simulink model "RBNN_NNT_NN_comparision_exp2"  (R2019a)
settings: Solver=FixedStepAuto  StartTime=0.0  StopTime=inf  FixedStep=0.0000001  RelTol=1e-3
libraries: dspstat3 x4, dsparch4 x2, simulink x1
settings Model: NumberOfSteps=16  Creator=vardhah  LastModifiedBy=vardhah
settings DataIOCC: ReturnWorkspaceOutputs=off
settings DebuggingCC: UnderSpecifiedDimensionMsg=warning  ArithmeticOperatorsInVariantConditions=warning

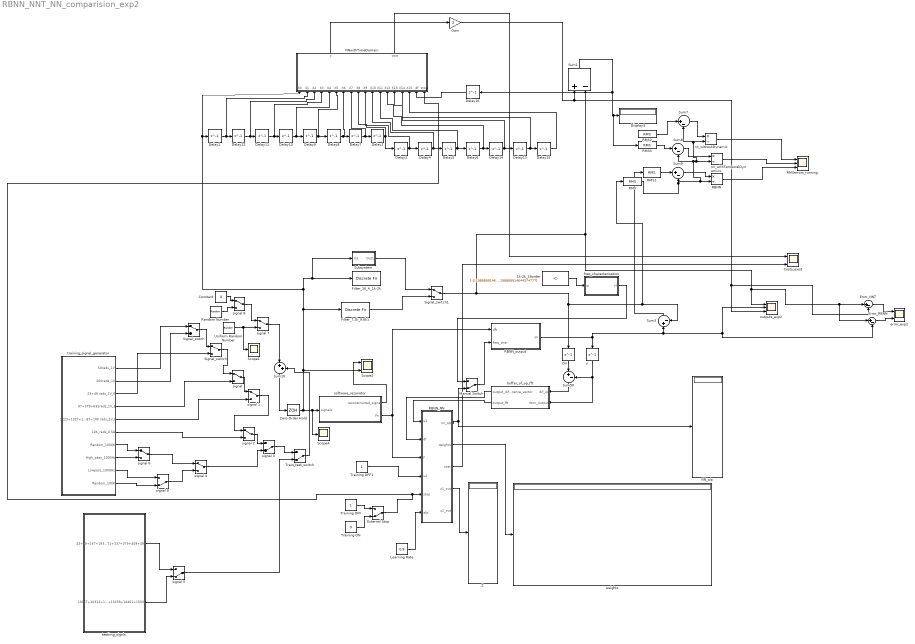
== system RBNN_NNT_NN_comparision_exp2 ==
  1k-2k_16order : Constant  Value=[-0.198889914644374777 0.0882189428518377339 0.0736891495871065116 0.0638368801789635787 0.0566372642221577294 0.0523172683654103132 0.0494565343907736044 0.048157521822162791 0.048157521822162791 0.0494565343907736044 0.0523172683654103132 0.0566372642221577294 0.0638368801789635787 0.0736891495871065116 0.0882189428518377339 -0.198889914644374777]  VectorParams1D=off
  Constant : Constant  Value=0
  Costs_exp2 : Scope  NumInputPorts=2
  Delay{1..16} (16 alike) : Delay  DelayLength=1  InitialCondition=0
  Display3 : Display
  Dn : Delay  DelayLength=1  InitialCondition=0
  Error_NNT : Sum  Inputs=|+-
  Error_RBNN : Sum  Inputs=|+-
  External Stop : ManualSwitch  CurrentSetting=0
  Filter_16_A_1k-2k : DiscreteFir  Tag=BlockMethodSubSystem  Coefficients=[-0.198889914644374777 0.0882189428518377339 0.0736891495871065116 0.0638368801789635787 0.0566372642221577294 0.0523172683654103132 0.0494565343907736044 0.048157521822162791 0.048157521822162791 0.0494565343907736044 0.0523172683654103132 0.0566372642221577294 0.0638368801789635787 0.0736891495871065116 0.0882189428518377339 -0.198889914644374777]  InputProcessing=Columns as channels (frame based)
  Filter_7.2k_9.6k1 : DiscreteFir  Tag=BlockMethodSubSystem  Coefficients=[-0.0120785049852322399 -0.0942455273574688279 0.0101245004695954266 0.125460404555770566 0.034165372769331126 -0.1614987160724079 -0.0984930555982914957 0.150982315564688691 0.150982315564688691 -0.0984930555982914957 -0.1614987160724079 0.034165372769331126 0.125460404555770566 0.0101245004695954266 -0.0942455273574688279 -0.0120785049852322399]  InputProcessing=Columns as channels (frame based)
  Gain : Gain  Gain=2
  Learning Rate : Constant  Value=0.9
  Manual Switch : ManualSwitch  CurrentSetting=0  varsize=on
  NN_o/p : Display
  NNwithTimeDomain : MATLAB Function  TreatAsAtomicUnit=on
  RBNN : Product  Inputs=*/
  RBNN_NN : MATLAB Function  TreatAsAtomicUnit=on
  RBNN_output : MATLAB Function  TreatAsAtomicUnit=on
  RMS{,1..3} (4 alike) : dspstat3/RMS  run=on  directionMode=Each column  dimension=1  InputProcessing=Columns as channels (frame based)  reset_popup=None
  RMSerrors_running : Scope  NumInputPorts=3
  Random Number : RandomNumber  Variance=0.1  SampleTime=0.000001
  Scope1 : Scope
  Scope2 : Scope  NumInputPorts=2
  Scope4 : Scope
  Signal_switch : ManualSwitch
  Signal_switch1 : ManualSwitch
  Signal_swtch : ManualSwitch
  Subsystem : Subsystem
  Sum1 : Sum  Inputs=+-
  Sum10 : Sum  Inputs=|++
  Sum{3,7..9,50} (5 alike) : Sum  Inputs=|+-
  Train_test_switch : ManualSwitch  CurrentSetting=0
  Training OFF : Constant
  Training OFF1 : Constant
  Training ON : Constant  Value=0
  Uniform Random Number : UniformRandomNumber  Minimum=-0.05  Maximum=0.05  SampleTime=0.000001
  Z : Display
  Zero-Order Hold : ZeroOrderHold  SampleTime=0.0000001
  buffer_of_op_fft : MATLAB Function  TreatAsAtomicUnit=on
  error_exp2 : Scope  NumInputPorts=2
  freq_characterisation : MATLAB Function  TreatAsAtomicUnit=on
  nn_withTemporalDynamics : Product  Inputs=*/
  nn_withoutDynamic : Product  Inputs=*/
  outputs_exp2 : Scope  NumInputPorts=3
  signal {,1..2,4,6..8} (7 alike) : ManualSwitch
  signal 3 : ManualSwitch  CurrentSetting=0
  signal 5 : ManualSwitch  CurrentSetting=0
  signal 9 : ManualSwitch  CurrentSetting=0
  software_rezonator : MATLAB Function  TreatAsAtomicUnit=on
  testimg_signls : Subsystem
  training_signal_generator : Subsystem
  weights : Display
  y : Delay  DelayLength=1  InitialCondition=0
  wires:
  software_rezonator/1(reconstructed_signal) -> Scope2/1
  software_rezonator/2(Fn) -> RBNN_output/1(dft), RBNN_NN/3(F)
  Dn/1 -> Sum50/1
  y/1 -> buffer_of_op_fft/2(rbnn_output), Sum50/2
  Manual Switch/1 -> RBNN_output/2(freq_char)
  freq_characterisation/1(H) -> Manual Switch/1
  RBNN_NN/1(nn_op) -> Manual Switch/2, NN_o/p/1
  External Stop/1 -> NNwithTimeDomain/18(stop), RBNN_NN/5(stop)
  Training OFF/1 -> External Stop/1
  Training ON/1 -> External Stop/2
  RBNN_NN/3(cost) -> Costs_exp2/2
  RBNN_NN/2(weights) -> weights/1
  RBNN_NN/4(z1_out) -> Z/1
  1k-2k_16order/1 -> freq_characterisation/1(ip)
  Sum50/1 -> buffer_of_op_fft/1(dif_ip)
  buffer_of_op_fft/1(output_difference_vector) -> RBNN_NN/2(df)
  buffer_of_op_fft/2(output_fft) -> RBNN_NN/1(u1)
  Training OFF1/1 -> RBNN_NN/4(u2)
  Signal_switch/1 -> "signal "/1
  Signal_swtch/1 -> Signal_switch/1
  "signal "/1 -> signal 1/1
  signal 1/1 -> signal 2/1
  training_signal_generator/4(97+379+631rads_1V_E) -> "signal "/2
  training_signal_generator/1(50rads_1V) -> Signal_swtch/1
  training_signal_generator/2(200rads_1V) -> Signal_swtch/2
  training_signal_generator/3(23+46 rads_1V_E) -> Signal_switch/2
  training_signal_generator/5(1223+1327+1637+1787+10K rads_1V_E) -> signal 1/2
  training_signal_generator/6(10K_rads_0.5A) -> signal 2/2
  signal 2/1 -> signal 3/1
  NNwithTimeDomain/1(y) -> Gain/1
  Delay16/1 -> NNwithTimeDomain/17(df)
  Delay4/1 -> NNwithTimeDomain/11(X10), Delay5/1
  Delay6/1 -> Delay14/1, NNwithTimeDomain/13(X12)
  Delay5/1 -> NNwithTimeDomain/12(X11), Delay6/1
  NNwithTimeDomain/2(cost) -> Costs_exp2/1
  Delay2/1 -> Delay3/1, NNwithTimeDomain/9(X8)
  Delay15/1 -> NNwithTimeDomain/16(X15)
  Delay13/1 -> NNwithTimeDomain/15(X14), Delay15/1
  Delay14/1 -> NNwithTimeDomain/14(X13), Delay13/1
  Delay10/1 -> NNwithTimeDomain/5(X4), Delay9/1
  Zero-Order Hold/1 -> Scope2/2, Subsystem/1(In1), Filter_16_A_1k-2k/1, NNwithTimeDomain/1(X0), Delay1/1, Filter_7.2k_9.6k1/1, Scope4/1, software_rezonator/1(signalz)
  Delay3/1 -> Delay4/1, NNwithTimeDomain/10(X9)
  Delay7/1 -> Delay2/1, NNwithTimeDomain/8(X7)
  Delay8/1 -> NNwithTimeDomain/7(X6), Delay7/1
  Delay1/1 -> NNwithTimeDomain/2(X1), Delay12/1
  Delay9/1 -> Delay8/1, NNwithTimeDomain/6(X5)
  Delay12/1 -> NNwithTimeDomain/3(X2), Delay11/1
  Delay11/1 -> Delay10/1, NNwithTimeDomain/4(X3)
  Sum1/1 -> RMS3/1, Display3/1, Delay16/1
  signal 4/1 -> signal 3/2
  Filter_7.2k_9.6k1/1 -> Signal_switch1/2
  nn_withoutDynamic/1 -> RMSerrors_running/1
  nn_withTemporalDynamics/1 -> RMSerrors_running/2
  RBNN/1 -> RMSerrors_running/3
  RMS/1 -> Sum7/2, nn_withoutDynamic/2, nn_withTemporalDynamics/2, Sum8/2, RBNN/2, Sum9/2
  Sum3/1 -> RMS1/1
  RMS1/1 -> Sum9/1
  RMS3/1 -> Sum8/1
  Sum8/1 -> nn_withTemporalDynamics/1
  RMS2/1 -> Sum7/1
  Sum7/1 -> nn_withoutDynamic/1
  testimg_signls/1(43+89+167+193+229+271+337+379+409+499) -> signal 5/1
  testimg_signls/2("10067+10313+10987+11299+11491+12161+12451+13259+14461+15031 ") -> signal 5/2
  signal 3/1 -> Train_test_switch/1
  signal 5/1 -> Train_test_switch/2
  Sum9/1 -> RBNN/1
  signal 7/1 -> Sum10/1
  Sum10/1 -> Zero-Order Hold/1
  Train_test_switch/1 -> Sum10/2
  Uniform Random Number/1 -> Scope1/1, signal 7/2
  Constant/1 -> signal 8/1
  signal 8/1 -> signal 7/1
  Random Number/1 -> signal 8/2
  Error_RBNN/1 -> error_exp2/2
  Gain/1 -> Error_NNT/2, outputs_exp2/3, Sum1/1
  Error_NNT/1 -> error_exp2/1
  Signal_switch1/1 -> Sum1/2, Error_RBNN/1, Error_NNT/1, outputs_exp2/1, RMS/1, Sum3/2, Dn/1
  RBNN_output/1(yn) -> Sum3/1, outputs_exp2/2, Error_RBNN/2, y/1
  signal 9/1 -> signal 4/2
  training_signal_generator/7(Random_1000K) -> signal 6/1
  training_signal_generator/8(High_pass_1000Hz) -> signal 6/2
  training_signal_generator/9(Lowpass_1000Hz) -> signal 9/1
  training_signal_generator/10(Random_100K) -> signal 9/2
  signal 6/1 -> signal 4/1
  Learning Rate/1 -> RBNN_NN/6(alp)
  Subsystem/1(Out1) -> Signal_switch1/1

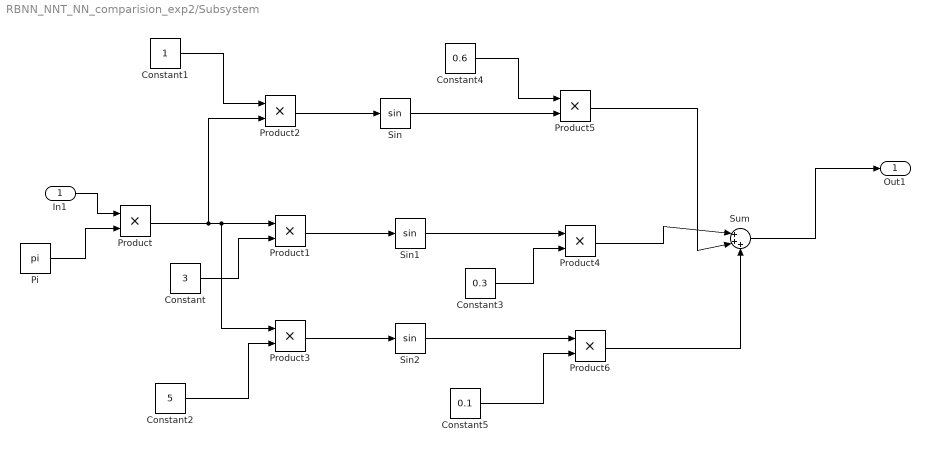
== system RBNN_NNT_NN_comparision_exp2/Subsystem ==
  In1 : Inport
  Constant : Constant  Value=3
  Constant1 : Constant
  Constant2 : Constant  Value=5
  Constant3 : Constant  Value=0.3
  Constant4 : Constant  Value=0.6
  Constant5 : Constant  Value=0.1
  Pi : Constant  Value=pi  OutDataTypeStr=Inherit: Inherit via back propagation
  Product{,1..6} (7 alike) : Product
  Sin : Trigonometry
  Sin1 : Trigonometry
  Sin2 : Trigonometry
  Sum : Sum  Inputs=|+++
  Out1 : Outport
  wires:
  Pi/1 -> Product/2
  In1/1 -> Product/1
  Constant1/1 -> Product2/1
  Product/1 -> Product2/2, Product3/1, Product1/1
  Constant/1 -> Product1/2
  Constant2/1 -> Product3/2
  Product2/1 -> Sin/1
  Product3/1 -> Sin2/1
  Product1/1 -> Sin1/1
  Product5/1 -> Sum/2
  Constant4/1 -> Product5/1
  Product6/1 -> Sum/3
  Constant5/1 -> Product6/2
  Constant3/1 -> Product4/2
  Product4/1 -> Sum/1
  Sin1/1 -> Product4/1
  Sin/1 -> Product5/2
  Sin2/1 -> Product6/1
  Sum/1 -> Out1/1

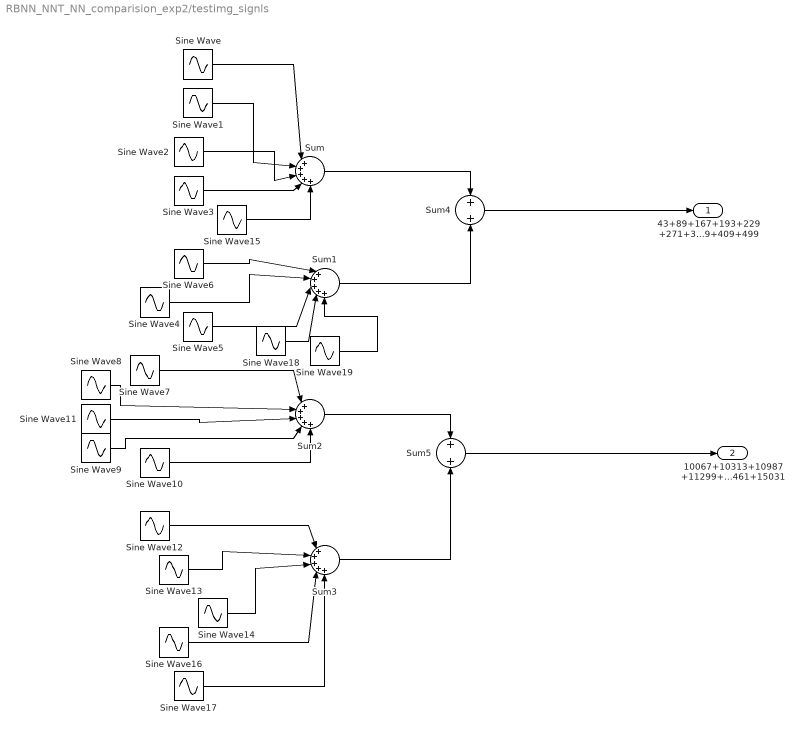
== system RBNN_NNT_NN_comparision_exp2/testimg_signls ==
  Sine Wave : Sin  Amplitude=0.1  Frequency=43  SampleTime=0
  Sine Wave1 : Sin  Amplitude=0.1  Frequency=89  SampleTime=0
  Sine Wave10 : Sin  Amplitude=0.1  Frequency=1491  SampleTime=0
  Sine Wave11 : Sin  Amplitude=0.1  Frequency=1987  SampleTime=0
  Sine Wave12 : Sin  Amplitude=0.1  Frequency=1261  SampleTime=0
  Sine Wave13 : Sin  Amplitude=0.1  Frequency=1451  SampleTime=0
  Sine Wave14 : Sin  Amplitude=0.1  Frequency=3359  SampleTime=0
  Sine Wave15 : Sin  Amplitude=0.1  Frequency=229  SampleTime=0
  Sine Wave16 : Sin  Amplitude=0.1  Frequency=2761  SampleTime=0
  Sine Wave17 : Sin  Amplitude=0.1  Frequency=2931  SampleTime=0
  Sine Wave18 : Sin  Amplitude=0.1  Frequency=409  SampleTime=0
  Sine Wave19 : Sin  Amplitude=0.1  Frequency=499  SampleTime=0
  Sine Wave2 : Sin  Amplitude=0.1  Frequency=167  SampleTime=0
  Sine Wave3 : Sin  Amplitude=0.1  Frequency=193  SampleTime=0
  Sine Wave4 : Sin  Amplitude=0.1  Frequency=337  SampleTime=0
  Sine Wave5 : Sin  Amplitude=0.1  Frequency=379  SampleTime=0
  Sine Wave6 : Sin  Amplitude=0.1  Frequency=271  SampleTime=0
  Sine Wave7 : Sin  Amplitude=0.1  Frequency=1067  SampleTime=0
  Sine Wave8 : Sin  Amplitude=0.1  Frequency=1313  SampleTime=0
  Sine Wave9 : Sin  Amplitude=0.1  Frequency=1299  SampleTime=0
  Sum{,1..3} (4 alike) : Sum  Inputs=|+++++
  Sum4 : Sum
  Sum5 : Sum
  43+89+167+193+229+271+337+379+409+499 : Outport
  "10067+10313+10987+11299+11491+12161+12451+13259+14461+15031 " : Outport  Port=2
  wires:
  Sine Wave4/1 -> Sum1/2
  Sine Wave5/1 -> Sum1/3
  Sine Wave6/1 -> Sum1/1
  Sine Wave7/1 -> Sum2/1
  Sine Wave8/1 -> Sum2/2
  Sine Wave11/1 -> Sum2/3
  Sine Wave9/1 -> Sum2/4
  Sine Wave10/1 -> Sum2/5
  Sine Wave/1 -> Sum/1
  Sine Wave1/1 -> Sum/2
  Sine Wave2/1 -> Sum/3
  Sine Wave3/1 -> Sum/4
  Sine Wave15/1 -> Sum/5
  Sine Wave17/1 -> Sum3/5
  Sine Wave16/1 -> Sum3/4
  Sine Wave14/1 -> Sum3/3
  Sine Wave13/1 -> Sum3/2
  Sine Wave12/1 -> Sum3/1
  Sine Wave18/1 -> Sum1/4
  Sine Wave19/1 -> Sum1/5
  Sum1/1 -> Sum4/2
  Sum/1 -> Sum4/1
  Sum4/1 -> 43+89+167+193+229+271+337+379+409+499/1
  Sum5/1 -> "10067+10313+10987+11299+11491+12161+12451+13259+14461+15031 "/1
  Sum2/1 -> Sum5/1
  Sum3/1 -> Sum5/2

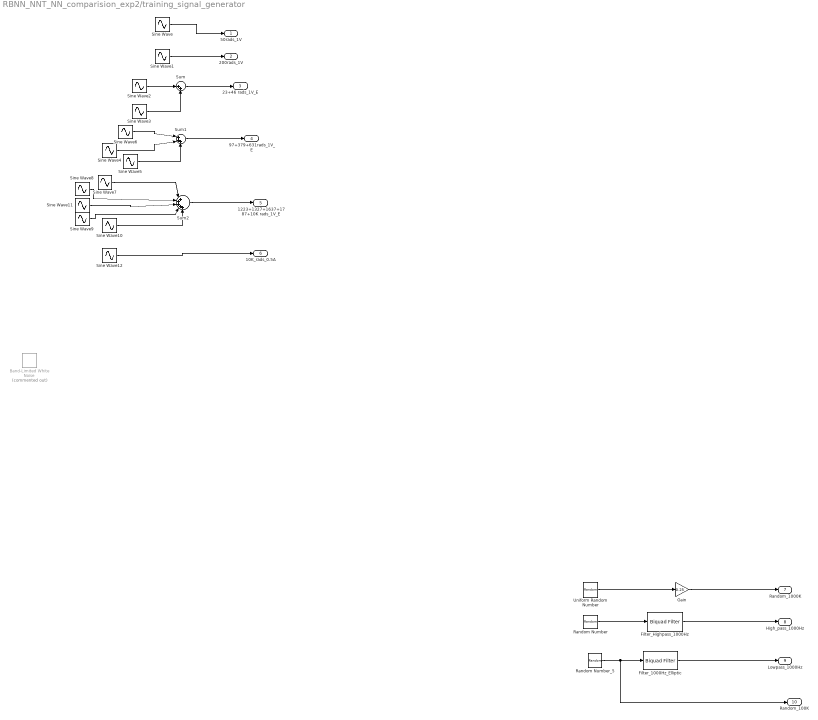
== system RBNN_NNT_NN_comparision_exp2/training_signal_generator ==
  Band-Limited White Noise : simulink/Sources/Band-Limited White Noise  Commented=on  Cov=[0.1]  Ts=0.1  seed=[23341]
  Filter_1000Hz_Elliptic : dsparch4/Biquad Filter  Tag=BlockMethodSubSystem  FilterSource=Dialog parameters  CoeffSource=Specify via dialog  FilterObject=BQF  IIRFiltStruct=Direct form II  BiQuadCoeffs=[1 -1.97632274641133088 1 1 -1.97939835930391728 0.996447647782941925;1 -1.97278944538463175 1 1 -1.97237302925889701 0.987301248342435933;1 -1.95955871016892758 1 1 -1.96235771308246942 0.972660421241710926;1 -1.88453112329299022 1 1 -1.95007892273323602 0.954154972801176005;1 1 0 1 -0.971866907997287366 0]  ScaleValues=[0.156742012624585314;0.548618699418480849;0.254757160374388947;0.035299988916345823;0.064621492680459483;1]  IC=0  ICnum=0  ICden=0  a0Flag=Warning  optimizeScaleValues=on  ScaleValueMode=Specify via input port (g)  InputProcessing=Columns as channels (frame based)  roundingMode=Floor  overflowMode=off  scaleValueFracLength=14  denProdOutputFracLength=30  denAccumFracLength=30  secondMemoryFracLength=15
      settings: SourceProductName=DSP System Toolbox
  Filter_Highpass_1000Hz : dsparch4/Biquad Filter  Tag=BlockMethodSubSystem  FilterSource=Dialog parameters  CoeffSource=Specify via dialog  FilterObject=BQF  IIRFiltStruct=Direct form II  BiQuadCoeffs=[1 -1.9832348135082305 1 1 -1.92871230100246671 0.962722433368264241;1 -1.98583197848424597 1 1 -1.86448430214602556 0.894880266245439038;1 -1.99020937824944788 1 1 -1.81348943480495617 0.839000119522318677;1 -1.99498360843622446 1 1 -1.77690733715439997 0.797591087467987903;1 -1.99863653257112794 1 1 -1.75501257669195576 0.772196386514157451;1 -1 0 1 -0.873867637211059756 0]  ScaleValues=[0.976953385016072651;0.943181897451958351;0.915362881516173843;0.894746706112661938;0.882102920451765637;0.936933818605529933;1]  IC=0  ICnum=0  ICden=0  a0Flag=Warning  optimizeScaleValues=on  ScaleValueMode=Specify via input port (g)  InputProcessing=Columns as channels (frame based)  roundingMode=Floor  overflowMode=off  scaleValueFracLength=14  denProdOutputFracLength=30  denAccumFracLength=30  secondMemoryFracLength=15
      settings: SourceProductName=DSP System Toolbox
  Gain : Gain  Gain=0.25
  Random Number : RandomNumber  Variance=0.5  SampleTime=0.000001
  Random Number_5 : RandomNumber  Variance=0.5  SampleTime=0.000001
  Sine Wave : Sin  Amplitude=0.8  Frequency=50  SampleTime=0
  Sine Wave1 : Sin  Frequency=200  SampleTime=0
  Sine Wave10 : Sin  Amplitude=0.2  Frequency=5000  SampleTime=0
  Sine Wave11 : Sin  Amplitude=0.2  Frequency=1637  SampleTime=0
  Sine Wave12 : Sin  Amplitude=0.5  Frequency=10000  SampleTime=0
  Sine Wave2 : Sin  Amplitude=0.5  Frequency=23  SampleTime=0
  Sine Wave3 : Sin  Amplitude=0.5  Frequency=46  SampleTime=0
  Sine Wave4 : Sin  Amplitude=0.33  Frequency=631  SampleTime=0
  Sine Wave5 : Sin  Amplitude=0.33  Frequency=379  SampleTime=0
  Sine Wave6 : Sin  Amplitude=0.33  Frequency=97  SampleTime=0
  Sine Wave7 : Sin  Amplitude=0.2  Frequency=1223  SampleTime=0
  Sine Wave8 : Sin  Amplitude=0.2  Frequency=1327  SampleTime=0
  Sine Wave9 : Sin  Amplitude=0.2  Frequency=1787  SampleTime=0
  Sum : Sum  Inputs=|++
  Sum1 : Sum  Inputs=|+++
  Sum2 : Sum  Inputs=|+++++
  Uniform Random Number : UniformRandomNumber  Minimum=-2  Maximum=2  SampleTime=0.0000002
  50rads_1V : Outport
  200rads_1V : Outport  Port=2
  23+46 rads_1V_E : Outport  Port=3
  97+379+631rads_1V_E : Outport  Port=4
  1223+1327+1637+1787+10K rads_1V_E : Outport  Port=5
  10K_rads_0.5A : Outport  Port=6
  Random_1000K : Outport  Port=7
  High_pass_1000Hz : Outport  Port=8
  Lowpass_1000Hz : Outport  Port=9
  Random_100K : Outport  Port=10
  wires:
  Sine Wave/1 -> 50rads_1V/1
  Sine Wave1/1 -> 200rads_1V/1
  Sine Wave2/1 -> Sum/1
  Sine Wave3/1 -> Sum/2
  Sum/1 -> 23+46 rads_1V_E/1
  Sine Wave4/1 -> Sum1/2
  Sine Wave5/1 -> Sum1/3
  Sine Wave6/1 -> Sum1/1
  Sum1/1 -> 97+379+631rads_1V_E/1
  Sine Wave7/1 -> Sum2/1
  Sine Wave8/1 -> Sum2/2
  Sine Wave11/1 -> Sum2/3
  Sine Wave9/1 -> Sum2/4
  Sine Wave10/1 -> Sum2/5
  Sum2/1 -> 1223+1327+1637+1787+10K rads_1V_E/1
  Sine Wave12/1 -> 10K_rads_0.5A/1
  Uniform Random Number/1 -> Gain/1
  Gain/1 -> Random_1000K/1
  Random Number/1 -> Filter_Highpass_1000Hz/1
  Filter_Highpass_1000Hz/1 -> High_pass_1000Hz/1
  Filter_1000Hz_Elliptic/1 -> Lowpass_1000Hz/1
  Random Number_5/1 -> Random_100K/1, Filter_1000Hz_Elliptic/1

== matlab function RBNN_NNT_NN_comparision_exp2/RBNN_NN ==
  settings: sampleTime=0.01
  data: u1 input; df input; F input; u2 input; stop input; nn_op output; alp input; weights output; cost output; z1_out output; z2_out output
function [nn_op,weights,cost,z1_out,z2_out]  = NN(u1,df,F,u2,stop,alp)

persistent w1 w2;
persistent vy;
persistent g1 g2;
persistent itr;
persistent J;
persistent del_w1 del_w2;
persistent mult1 mult2 ;
persistent memory_alloc_flag;
persistent n;

%%
%%%%%%----------------------------------------------------------------------------%%%%%
%Hyper-parameter & other tunable part of code

M=1;   %declare batch size of training (It will also be equal to number of input in our case as we are using DFT)
E=1;    % size of external associative input

%layer declaration
layer_1=16;
layer_2=16;

%learning rate. Currently reading from input pin 
alpha = alp;

%others
input_layer =M+E;       %layer_0
output_layer=layer_2;

% weight Intialisation 
if isempty(w1)
       w1=randn(input_layer,layer_1)*0.1;
end
if isempty(w2)
       w2=randn(layer_1,layer_2)*0.1;
end


%%%%%---------------------------------------------------------------------------------%%%%%

%%

%synchronising clock
if isempty(n)
        n = 0; end
n=n+1;

%%
%Allocation of variables that will be used during runtime( one time execution code) 
if isempty(memory_alloc_flag)
        memory_alloc_flag = 0; 
end
if isempty(mult1)
       mult1=zeros(layer_1,layer_1*input_layer); 
end
if isempty(mult2)
       mult2=zeros(layer_2,layer_1*layer_2); 
end

if isempty(vy)
       vy=zeros(input_layer,M); 
end

if memory_alloc_flag==0
 %write memory allocation for looped code here.It runs once and store it in memory.  
 mult1=[];
 mult2=[];
  for iteration =1:layer_1
   mult1=[mult1;[zeros(1,(iteration-1)*input_layer) ones(1,input_layer) zeros(1,(layer_1-iteration)*input_layer)]];
  end
  for iterate=1:layer_2
   mult2=[mult2;[zeros(1,(iterate-1)*layer_1) ones(1,layer_1) zeros(1,(layer_2-iterate)*layer_1)]];
  end
  
 for k= 1:input_layer
    for j = 1:M 
        if k<=(M/2)+1 && k>=1
            vy(k,j)=(1/M)*cos(pi*(M-j)*(k-1)/(M/2));
        elseif k<=M && k>=(M/2)+1
            vy(k,j)=-(1/M)*sin(pi*(M-j)*(k-1)/(M/2));
        elseif k>M
            vy(k,j)=0;     
        end
    end
 end
 memory_alloc_flag=1; 
end

%%
%============All other Initiaisation =========================>

%Initialisation of delta of weight storage
if isempty(del_w1)
    del_w1=zeros(1,input_layer*layer_1);
end
if isempty(del_w2)
    del_w2=zeros(1,layer_2*layer_1);
end


%Intialising iteration number & cost value. 
if isempty(itr)
    itr=0;
end
if isempty(J)
    J=0;
end


%gradient initialisation(in matrix form)
if isempty(g1)
    g1= zeros(M,input_layer*layer_1);   
end
if isempty(g2)
    g2= zeros(M,layer_1*layer_2);   
end


%%
%Input vector creation code block
x_in = [real(u1(1:(size(u1,2)/2)+1)) imag(u1(1:(size(u1,2)/2)-1))];
v=transpose([x_in transpose(u2)]);

%%
%RBNN core vectorised algorithm implementation 

%--------------->forward propogation ------------>

z1=w1'*v ;
a1=(1./(1+exp(-z1)));
an1=(a1-0.5);
z2=w2'*an1 ;
a2=(1./(1+exp(-z2)));
an2=(a2-0.5);

%-------------> Backward Propogation -------->

%calculation of Nv:
da2_z2=a2.*(1-a2);
dn_a1=w2'.*repmat(da2_z2,1,layer_1);
%da2_z2=a2.*(1-a2);
%dn_z2= dn_a2.* repmat(transpose(da2_z2),output_layer,1);
%dn_a1=dn_z2*w2';
da1_z1=a1.*(1-a1); 
dn_z1=dn_a1.*repmat(transpose(da1_z1),output_layer,1);
dn_v=dn_z1*w1';   %"This is Nv" 

%calculation of aD, A & B 
aD=transpose(F)*dn_v*vy;
A=[aD;eye(M-1) zeros(M-1,1)];
B=[transpose(F) ; zeros(M-1,size(F,1))]; 

%calculation of Nw(diff of N(v,w) wrt each weights)
dIn_2= da2_z2*transpose(a1);
dn_w2=repmat(dIn_2,1,layer_2).* mult2;

%dIn_2= da2_z2*transpose(a1);
%da2_w2=repmat(dIn_2,1,layer_2).* mult2;
%dn_w2=dn_a2*da2_w2;

dIn_1= da1_z1*transpose(v);
da1_w1= repmat(dIn_1,1,layer_1).*mult1;
dn_w1=dn_a1*da1_w1;

%gradient updation
%g3=A*g3+B*dn_w3;
g2=A*g2+B*dn_w2;
g1=A*g1+B*dn_w1;

%Training & updation only once in a batch(batch size=M,n=Overall counter) 
if mod(n,M)==0 && stop==0
    del_w1 =alpha*df*1*g1/M ;
    del_w2 =alpha*df*1*g2/M ;
    %del_w3 =alpha*df*1*g3/M ;
    del_w_reshaped1= reshape(del_w1,[input_layer,layer_1]);
    del_w_reshaped2= reshape(del_w2,[layer_1,layer_2]);
    %del_w_reshaped3= reshape(del_w3,[layer_2,layer_3]);
    w1=w1+ del_w_reshaped1;
    w2=w2+ del_w_reshaped2;
    %w3=w3+ del_w_reshaped3; 
    itr=itr+1;
   
end
 J= sum(df.^2,'all')/(2*M);
%For logging & visulisation purpose
cost=J;
weights=w1;
z1_out=z1;
z2_out=z2;

%NN output assignment
nn_op=an2;


end

== matlab function RBNN_NNT_NN_comparision_exp2/buffer_of_op_fft ==
  data: output_difference_vector output size=[1,16]; output_fft output size=[1,16]; dif_ip input; rbnn_output input
function [output_difference_vector,output_fft] = difBuffer(dif_ip,rbnn_output)                      

 sz=4;                       % size of the dft 
 
 persistent a;
 persistent b;
 if isempty(b)
  b= zeros(1,sz);
 end
 if isempty(a)
  a= zeros(1,sz);
 end
 
 
  a= circshift(a,1);
  a(1)=dif_ip;
  b= circshift(b,1);
  b(1)=rbnn_output;

 output_difference_vector=a; 
 output_fft=1/sz*fft(b); 
end

== matlab function RBNN_NNT_NN_comparision_exp2/freq_characterisation ==
  data: ip input; H output
function H  = freq_character(ip)                      

dft_of_ip=fft(ip); 
size_dft=size(dft_of_ip,2)/2;
H =transpose([real(dft_of_ip(1:size_dft+1)) imag(dft_of_ip(2:size_dft))]);

end

== matlab function RBNN_NNT_NN_comparision_exp2/NNwithTimeDomain ==
  settings: sampleTime=0.125
  data: X0 input; X1 input; X2 input; X3 input; X4 input; X5 input; X6 input; X7 input; X8 input; X9 input; X10 input; X11 input; X12 input; X13 input; X14 input; X15 input; df input; y output; cost output; stop input
function [y,cost] = NN(X0,X1,X2,X3,X4,X5,X6,X7,X8,X9,X10,X11,X12,X13,X14,X15,df,stop)

%This is a generalised code for 2 layer - multiple input-single output network.
% to alter the network (1) "change layer's size" in layer declaration below (2) the function
%input and output above and (3) Input matrix creation. (4) change inputs in
%simulink design

alpha = 0.001;

%(1)layer decalration
layer_0= 16;
layer_1= 16;
layer_2 =16;
layer_3=1;
M=2;

%(2) is above in function block

%(3)parameter intialisation
v=[X0 X1 X2 X3 X4 X5 X6 X7 X8 X9 X10 X11 X12 X13 X14 X15];

%Do not alter the code below. The below implementaion is generalised for
%multiple input and single output, 2 layer neural network. 


persistent w1 w2 w3;
persistent a1 a2 a3;
persistent J; 
persistent v_old n; 

if isempty(a1)
    a1= zeros(layer_1,1);
end

if isempty(a2)
    a2= zeros(layer_2,1);
end
if isempty(a3)
    a3= zeros(layer_3,1);
end

if isempty(J)
    J= 0;
end
if isempty(v_old)
    v_old= zeros(1,layer_0);
end

if isempty(w1)
       w1=randn(layer_1,layer_0);
end
if isempty(w2)
       w2=randn(layer_2,layer_1);
end
if isempty(w3)
       w3=randn(layer_3,layer_2);
end

%synchronising clock
if isempty(n)
        n = 0; end
n=n+1;



%BackProp:
if mod(n,M)==0 && stop==0
 dz3=a3.*(1-a3)*df*-1;
 dw3=dz3*transpose(a2);
 dz2=(a2.*(1-a2)).*(w3'*dz3);
 dw2=dz2*transpose(a1);
 dz1=(a1.*(1-a1)).*(w2'*dz2);
 dw1=dz1*v;
 w3=w3 + alpha*dw3;
 w2=w2 + alpha*dw2;
 w1=w1 + alpha*dw1;
 v_old=v;
end 

%forward propogation
z1=w1*v';
a1= (1./(1+exp(-z1)));
an1=a1-0.5;
z2=w2*an1;
a2= (1./(1+exp(-z2)));
an2=a2-0.5;
z3=w3*an2;
a3= (1./(1+exp(-z3)));
an3=a3-0.5;
cost=1/2*df^2;

%output assignment
y=an3;


end

== matlab function RBNN_NNT_NN_comparision_exp2/software_rezonator ==
  data: signalz input; reconstructed_signal output; Fn output size=16
function [reconstructed_signal,Fn]   = rezonator(signalz)

persistent numberofrezonator;
persistent g c bfr_rezo_sm aft_delay dft_out;
persistent out signal_dif;
persistent n;
persistent memory_alloc_flag;


%assign the number of rezonator here. For configuring it for higher order
%rezonator  we need to change (1) 'numberofrezonaotor' variable
if isempty(numberofrezonator)
        numberofrezonator = 16;   %here 16 parallel rezonators
end

%Initialisation of memory allocations/variables ====> 
if isempty(memory_alloc_flag)
        memory_alloc_flag = 0; 
end
if isempty(g)
       g=zeros(numberofrezonator,numberofrezonator,'like',0i); 
end
if isempty(c)
       c=zeros(numberofrezonator,numberofrezonator,'like',0i); 
end
if memory_alloc_flag==0
 for i=0:numberofrezonator-1
  for j= 0:numberofrezonator-1
   g(i+1,j+1)=1/numberofrezonator*(exp(-1i*2*pi*i*j/numberofrezonator));
   c(i+1,j+1)=(exp(1i*2*pi*i*j/numberofrezonator));
  end 
 end
 memory_alloc_flag=1;
end


%Initialisation of variables  =====> 
if isempty(n)
        n = 0;   
end 
if isempty(out)
  out=0+0i;
end
if isempty(signal_dif)
  signal_dif=0+0i;
end
if isempty(bfr_rezo_sm)
  bfr_rezo_sm=repmat(0+0i,numberofrezonator,1);
end
if isempty(aft_delay)
  aft_delay=repmat(0+0i,numberofrezonator,1);
end
if isempty(dft_out)
  dft_out=repmat(0+0i,numberofrezonator,1);
end

%creating cycle of rotation for selection of correct column of g & c.
cycle=mod(n,numberofrezonator);

%resonator core -----------------------------> 
dft_out=c(:,cycle+1).*aft_delay;
out= sum(dft_out,1);
signal_dif=signalz-out;
bfr_rezo_sm=g(:,cycle+1).*signal_dif;

%counting the counter
n=n+1;

% output assignment ------------------>
reconstructed_signal=out;
dft=aft_delay; 
N=size(dft,1);
a=1:1:N/2-1;
b=N/2+1:1:N-1;
dft_trans=transpose(dft);
Fn=transpose([real(dft_trans(1)) 2*(real(dft_trans(2:N/2)).*cos(2*pi*a*n/N)-imag(dft_trans(2:N/2)).*sin(2*pi*a*n/N)) -1^n*real(dft_trans(N/2+1)) -2*(imag(dft_trans(N/2+2:N)).*cos(2*pi*b*n/N)+real(dft_trans(N/2+2:N)).*sin(2*pi*b*n/N))]);
%--------output assignment over----------<

%final updation of buffer ------>>>>>>>>>>>>
aft_delay= aft_delay+bfr_rezo_sm; 
end

== matlab function RBNN_NNT_NN_comparision_exp2/RBNN_output ==
  data: dft input; yn output; freq_char input
function yn = fcn(dft,freq_char)
yn=transpose(freq_char)*dft;
end
